simulink model "soal_2"  (R2021b)
settings: Solver=VariableStepAuto  StartTime=0.0  StopTime=10.0  RelTol=1e-3
settings Model: Creator=nnxvnx  LastModifiedBy=Arya

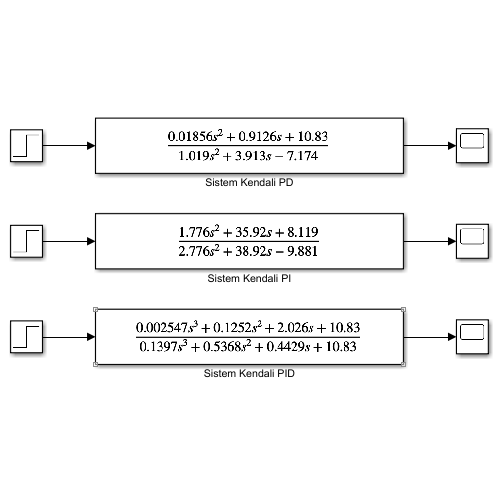
[thumbnail: Simulink's stored preview of the top-level diagram]
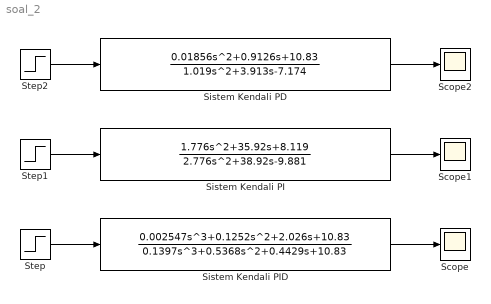
== system soal_2 ==
  Scope : Scope
  Scope1 : Scope
  Scope2 : Scope
  Sistem Kendali PD : TransferFcn  Numerator=[0.01856 0.9126 10.83]  Denominator=[1.019 3.913 -7.174]
  Sistem Kendali PI : TransferFcn  Numerator=[1.776 35.92 8.119]  Denominator=[2.776 38.92 -9.881]
  Sistem Kendali PID : TransferFcn  Numerator=[0.002547 0.1252 2.026 10.83]  Denominator=[0.1397 0.5368 0.4429 10.83]
  Step : Step  SampleTime=0
  Step1 : Step  SampleTime=0
  Step2 : Step  SampleTime=0
  wires:
  Step/1 -> Sistem Kendali PID/1
  Sistem Kendali PID/1 -> Scope/1
  Sistem Kendali PI/1 -> Scope1/1
  Step1/1 -> Sistem Kendali PI/1
  Step2/1 -> Sistem Kendali PD/1
  Sistem Kendali PD/1 -> Scope2/1
